simulink model "cyclocopter"  (R2015b)
settings: Solver=VariableStepAuto  SolverMode=SingleTasking  StartTime=0.0  StopTime=100  FixedStep=0.001  RelTol=1e-3
InitFcn:
  | % Update Rates, 50Hz for RC kit
  | fs_servo = 50; %Hz
  | Ts_servo = 1/fs_servo;
  | 
  | % Rates of changes
  | rate = 500; % rad/s per second change
  | rate_p = 2000; % Same for balancing props
  | 
  | % Motor limits
  | limit_high = 8000 * (2 * pi / 60); % rad/s
  | limit_low = 300 * (2 * pi / 60); % rad/s
  | 
  | limit_p_high = 20000 * (2 * pi / 60); % rad/s
  | limit_p_low  = 2000 * (2 * pi / 60);
  | 
  | % Eccentric point limits
  | servo_offset = 0.22;
  | servo_high = pi/4 + servo_offset; %45 deg
  | servo_low = -pi/4 + servo_offset; %45 deg
  | 
  | % Controller Update rate
  | fs = 200; % Hz
  | Ts = 1/fs;
  | 
  | % Constantss
  | g = 9.81; % Gravity
  | 
  | load('cyclorotor_lookup.mat');
values from neighbouring files (symbols this model uses):
  breakpoint_epsilon = [0 0.0175019089336 0.0350038178673 0.0525057268009 0.0700076357346 0.0875095446682 0.105011453602 0.122513362536 0.140015271469 0.157517180403 0.175019089336 0.19252099827 ... (360 elements, 1x360)]    [cyclorotor_lookup.mat]
  breakpoint_omega = [0 5.26229925224 10.5245985045 15.7868977567 21.049197009 26.3114962612 31.5737955135 36.8360947657 42.098394018 47.3606932702 52.6229925224 57.8852917747 ... (200 elements, 1x200)]    [cyclorotor_lookup.mat]
  cyclorotor_lookup = [0 -0.000183077012455 -0.000732308049818 -0.00164769311209 -0.00292923219927 -0.00457692531136 -0.00659077244836 -0.00897077361027 -0.0117169287971 -0.0148292380088 -0.0183077012455 -0.022152318507 ... (432000 elements, 200x360x6)]    [cyclorotor_lookup.mat]
  F = zeros(3, numPoints)    [test_cyclorotor.m]
  r = 0.069    [Cyclorotor.m]
undefined symbols (not defined in the file or in its folder): MIL
libraries: simulink x14, aerolibwind2 x1, aerolibtransform2 x1
settings Model: Creator=freddiesherratt  LastModifiedBy=freddiesherratt
settings DataIOCC: MaxDataPoints=4000  SaveOutput=off  SaveTime=off

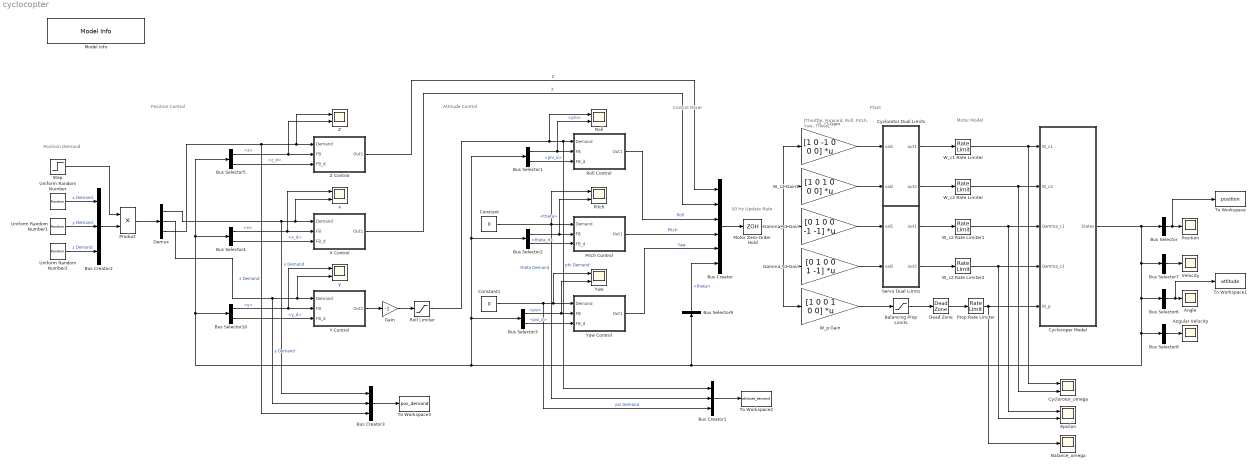
== system cyclocopter ==
  note: Position Demand
  note: Attitude Control
  note: Plant
  note: 50 Hz Update Rate
  note: Motor Model
  note: Control Mixer
  note: [Throttle, Forward, Roll, Pitch, Yaw, Theta]
  note: Position Control
  Angle : Scope
  Angular Velocity : Scope
  Balance_omega : Scope
  Balancing Prop Limits : Saturate  UpperLimit=limit_p_high  LowerLimit=0
  Bus Creator : BusCreator  Inputs=6
  Bus Creator1 : BusCreator  Inputs=3
  Bus Creator2 : BusCreator  Inputs=3
  Bus Creator3 : BusCreator  Inputs=3
  Bus Selector : BusSelector  OutputSignals=x,y,z  OutputAsBus=on
  Bus Selector1 : BusSelector  OutputSignals=phi,phi_d
  Bus Selector10 : BusSelector  OutputSignals=y,y_d
  Bus Selector2 : BusSelector  OutputSignals=theta,theta_d
  Bus Selector3 : BusSelector  OutputSignals=psi,psi_d
  Bus Selector4 : BusSelector  OutputSignals=x,x_d
  Bus Selector5 : BusSelector  OutputSignals=z,z_d
  Bus Selector6 : BusSelector  OutputSignals=phi,theta,psi  OutputAsBus=on
  Bus Selector7 : BusSelector  OutputSignals=x_d,y_d,z_d  OutputAsBus=on
  Bus Selector8 : BusSelector  OutputSignals=phi_d,theta_d,psi_d  OutputAsBus=on
  Bus Selector9 : BusSelector  OutputSignals=theta
  Constant : Constant  Value=0
  Constant1 : Constant  Value=0
  Cyclocoper Model : Subsystem  mask{Ic=0, Im=0, ws=4.5}
      mask prompts: Ic "Ic, Cyclorotor Inertia"; Im "Im, Motor inertia"; ws "ws, wind speed (m/s)"
  Cyclorotor Dual Limits : MATLAB Function  TreatAsAtomicUnit=on  mask{LL=limit_low, UL=limit_high}
      mask prompts: LL "LL, Lower Limit"; UL "UL, Upper Limit"
  Cyclorotor_omega : Scope  NumInputPorts=2
  Dead Zone : DeadZone  LowerValue=0  UpperValue=limit_p_low  SaturateOnIntegerOverflow=on
  Demux : Demux  Outputs=3
  Epsilon : Scope  NumInputPorts=2
  Gain : Gain  Gain=-1
  Gamma_c1 Gain : Gain  Gain=[0 1 0 0 -1 -1]  Multiplication=Matrix(K*u)
  Gamma_c2 Gain : Gain  Gain=[0 1 0 0 1 -1]  Multiplication=Matrix(K*u)
  Model Info : simulink/Model-Wide Utilities/Model Info  Frame=on  DisplayStringWithTags=|  HorizontalTextAlignment=Left  LeftAlignmentValue=0.02  SourceBlockDiagram=cyclocopter  TagMaxNumber=20
      | Last Modified: %<ModifiedDate>
      | By: %<LastModifiedBy>
      | version: %<ModelVersion>
  Motor Zero-Order Hold : ZeroOrderHold  SampleTime=Ts_servo
  Pitch : Scope  NumInputPorts=2
  Pitch Control : Subsystem  mask{P1=18, I1=0, D1=10, P2=25, I2=10, D2=20}
  Position : Scope
  Product : Product
  Prop Rate Limiter : RateLimiter  RisingSlewLimit=rate_p  FallingSlewLimit=-rate_p  SampleTimeMode=inherited  InitialCondition=50
  Roll : Scope  NumInputPorts=2
  Roll Control : Subsystem  mask{P1=10, I1=0, D1=10, P2=7, I2=0.2, D2=0.25}
  Roll Limiter : Saturate  UpperLimit=pi/3  LowerLimit=-pi/3
  Servo Dual Limits : MATLAB Function  TreatAsAtomicUnit=on  mask{LL=servo_low, UL=servo_high}
      mask prompts: LL "LL, Lower Limit"; UL "UL, Upper Limit"
  Step : Step  Time=20  SampleTime=0
  To Workspace : ToWorkspace  VariableName=position  SaveFormat=Timeseries  SampleTime=-1
  To Workspace1 : ToWorkspace  VariableName=attitude  SaveFormat=Timeseries  SampleTime=-1
  To Workspace2 : ToWorkspace  VariableName=attitude_demand  SaveFormat=Timeseries  SampleTime=-1
  To Workspace3 : ToWorkspace  VariableName=pos_demand  SaveFormat=Timeseries  SampleTime=-1
  Uniform Random Number : UniformRandomNumber  Minimum=-3  Maximum=3  SampleTime=10
  Uniform Random Number1 : UniformRandomNumber  Minimum=-3  Maximum=3  Seed=1  SampleTime=10
  Uniform Random Number2 : UniformRandomNumber  Minimum=-3  Maximum=3  Seed=2  SampleTime=10
  Velocity : Scope
  W_c1 Gain : Gain  Gain=[1 0 -1 0 0 0]  Multiplication=Matrix(K*u)
  W_c1 Rate Limiter : RateLimiter  RisingSlewLimit=rate  FallingSlewLimit=-rate
  W_c2 Gain1 : Gain  Gain="[1 0 1  0 0 0]"  Multiplication=Matrix(K*u)
  W_c2 Rate Limiter : RateLimiter  RisingSlewLimit=rate  FallingSlewLimit=-rate
  W_c2 Rate Limiter1 : RateLimiter  RisingSlewLimit=pi  FallingSlewLimit=-pi  InitialCondition=servo_offset
  W_c2 Rate Limiter2 : RateLimiter  RisingSlewLimit=pi  FallingSlewLimit=-pi  InitialCondition=servo_offset
  W_p Gain : Gain  Gain=[1 0 0 1 0 0]  Multiplication=Matrix(K*u)
  X Control : Subsystem  mask{P1=3.2, I1=0, D1=4, P2=0.8, I2=0.2, D2=0.3}
  Y Control : Subsystem  mask{P1=0.2, I1=0, D1=0.55, P2=0.5, I2=0.05, D2=0.15}
  Yaw : Scope  NumInputPorts=2
  Yaw Control : Subsystem  mask{P1=2, I1=0, D1=2, P2=0.4, I2=0.01, D2=0.03}
  Z : Scope  NumInputPorts=2
  Z Control : Subsystem  mask{P1=15, I1=0, D1=15, P2=2.8, I2=1.8, D2=1}
  x : Scope  NumInputPorts=2
  y : Scope  NumInputPorts=2
  wires:
  Bus Selector/1 -> Position/1, To Workspace/1
  Cyclorotor Dual Limits/2(out2) -> W_c2 Rate Limiter/1
  Cyclorotor Dual Limits/1(out1) -> W_c1 Rate Limiter/1
  Motor Zero-Order Hold/1 -> W_c1 Gain/1, W_c2 Gain1/1, W_p Gain/1, Gamma_c2 Gain/1, Gamma_c1 Gain/1
  Bus Creator/1 -> Motor Zero-Order Hold/1
  Roll Control/1(Out1) -> Bus Creator/3  "Roll"
  Z Control/1(Out1) -> Bus Creator/1  "Z"
  Gamma_c1 Gain/1 -> Servo Dual Limits/1(val1)
  Gamma_c2 Gain/1 -> Servo Dual Limits/2(val2)
  Yaw Control/1(Out1) -> Bus Creator/5  "Yaw"
  Pitch Control/1(Out1) -> Bus Creator/4  "Pitch"
  W_c2 Gain1/1 -> Cyclorotor Dual Limits/2(val2)
  W_c1 Gain/1 -> Cyclorotor Dual Limits/1(val1)
  X Control/1(Out1) -> Bus Creator/2  "X"
  Bus Selector5/1 -> Z/2, Z Control/2(FB)  "<z>"
  Bus Selector5/2 -> Z Control/3(FB_d)  "<z_d>"
  Bus Selector4/1 -> x/1, X Control/2(FB)  "<x>"
  Bus Selector4/2 -> X Control/3(FB_d)  "<x_d>"
  Bus Selector1/1 -> Roll/2, Roll Control/2(FB)  "<phi>"
  Bus Selector1/2 -> Roll Control/3(FB_d)  "<phi_d>"
  Bus Selector2/1 -> Pitch/2, Pitch Control/2(FB)  "<theta>"
  Bus Selector2/2 -> Pitch Control/3(FB_d)  "<theta_d>"
  Bus Selector3/1 -> Yaw/2, Yaw Control/2(FB)  "<psi>"
  Bus Selector3/2 -> Yaw Control/3(FB_d)  "<psi_d>"
  Demux/3 -> Bus Creator3/3, Z/1, Z Control/1(Demand)  "z Demand"
  Demux/1 -> Bus Creator3/1, x/2, X Control/1(Demand)  "x Demand"
  Constant/1 -> Pitch/1, Bus Creator1/2, Pitch Control/1(Demand)  "theta Demand"
  Constant1/1 -> Bus Creator1/3, Yaw/1, Yaw Control/1(Demand)  "psi Demand"
  W_c2 Rate Limiter/1 -> Cyclorotor_omega/2, Cyclocoper Model/2(W_c2)
  W_c1 Rate Limiter/1 -> Cyclorotor_omega/1, Cyclocoper Model/1(W_c1)
  Bus Selector6/1 -> Angle/1, To Workspace1/1
  Cyclocoper Model/1(States) -> Bus Selector10/1, Bus Selector4/1, Bus Selector5/1, Bus Selector1/1, Bus Selector2/1, Bus Selector3/1, Bus Selector9/1, Bus Selector8/1, Bus Selector6/1, Bus Selector7/1, Bus Selector/1
  Bus Selector7/1 -> Velocity/1
  Bus Selector8/1 -> Angular Velocity/1
  Bus Selector9/1 -> Bus Creator/6  "<theta>"
  Bus Selector10/1 -> y/1, Y Control/2(FB)  "<y>"
  Bus Selector10/2 -> Y Control/3(FB_d)  "<y_d>"
  Demux/2 -> Bus Creator3/2, y/2, Y Control/1(Demand)  "y Demand"
  Y Control/1(Out1) -> Gain/1
  Gain/1 -> Roll Limiter/1
  Balancing Prop Limits/1 -> Dead Zone/1
  Servo Dual Limits/1(out1) -> W_c2 Rate Limiter1/1
  Servo Dual Limits/2(out2) -> W_c2 Rate Limiter2/1
  W_p Gain/1 -> Balancing Prop Limits/1
  W_c2 Rate Limiter1/1 -> Epsilon/1, Cyclocoper Model/3(Gamma_c1)
  W_c2 Rate Limiter2/1 -> Epsilon/2, Cyclocoper Model/4(Gamma_c2)
  Roll Limiter/1 -> Roll/1, Bus Creator1/1, Roll Control/1(Demand)  "phi Demand"
  Dead Zone/1 -> Prop Rate Limiter/1
  Uniform Random Number2/1 -> Bus Creator2/3  "z Demand"
  Uniform Random Number1/1 -> Bus Creator2/2  "y Demand"
  Uniform Random Number/1 -> Bus Creator2/1  "x Demand"
  Bus Creator2/1 -> Product/2
  Step/1 -> Product/1
  Prop Rate Limiter/1 -> Balance_omega/1, Cyclocoper Model/5(W_p)
  Product/1 -> Demux/1
  Bus Creator1/1 -> To Workspace2/1
  Bus Creator3/1 -> To Workspace3/1

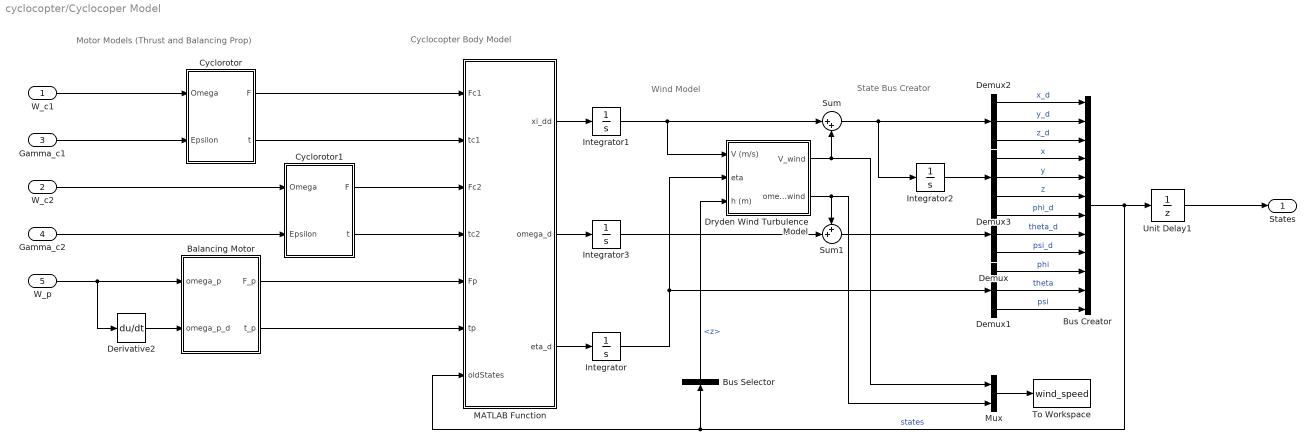
== system cyclocopter/Cyclocoper Model ==
  note: Wind Model
  note: State Bus Creator
  note: Cyclocopter Body Model
  note: Motor Models (Thrust and Balancing Prop)
  W_c1 : Inport
  W_c2 : Inport  Port=2
  Gamma_c1 : Inport  Port=3
  Gamma_c2 : Inport  Port=4
  W_p : Inport  Port=5
  Balancing Motor : MATLAB Function  TreatAsAtomicUnit=on  mask{I_m=Im}
  Bus Creator : BusCreator  Inputs=12
  Bus Selector : BusSelector  OutputSignals=z
  Cyclorotor : Subsystem  mask{I_c=Ic}
      mask prompts: I_c "I_c, Cyclorotor Rotational Inertia"
  Cyclorotor1 : Subsystem  mask{I_c=Ic}
      mask prompts: I_c "I_c, Cyclorotor Rotational Inertia"
  Demux{,1..3} (4 alike) : Demux  Outputs=3
  Derivative2 : Derivative
  Dryden Wind Turbulence Model : Subsystem  mask{ws=ws}
      mask prompts: ws "ws, wind speed (m/s)"
  Integrator{,1..3} (4 alike) : Integrator
  MATLAB Function : MATLAB Function  TreatAsAtomicUnit=on
  Mux : Mux  Inputs=2
  Sum : Sum  Inputs=|++
  Sum1 : Sum  Inputs=++|
  To Workspace : ToWorkspace  VariableName=wind_speed  SaveFormat=Timeseries  SampleTime=-1
  Unit Delay1 : UnitDelay  SampleTime=Ts
  States : Outport
  wires:
  Demux/3 -> Bus Creator/9  "psi_d"
  Demux1/1 -> Bus Creator/10  "phi"
  Balancing Motor/1(F_p) -> MATLAB Function/5(Fp)
  Bus Creator/1 -> Bus Selector/1, MATLAB Function/7(oldStates), Unit Delay1/1  "states"
  Demux3/2 -> Bus Creator/5  "y"
  Demux3/3 -> Bus Creator/6  "z"
  Demux/2 -> Bus Creator/8  "theta_d"
  Demux2/3 -> Bus Creator/3  "z_d"
  Demux3/1 -> Bus Creator/4  "x"
  Demux2/2 -> Bus Creator/2  "y_d"
  Demux2/1 -> Bus Creator/1  "x_d"
  Demux1/3 -> Bus Creator/12  "psi"
  Demux/1 -> Bus Creator/7  "phi_d"
  Demux1/2 -> Bus Creator/11  "theta"
  W_p/1 -> Derivative2/1, Balancing Motor/1(omega_p)
  Gamma_c2/1 -> Cyclorotor1/2(Epsilon)
  W_c2/1 -> Cyclorotor1/1(Omega)
  Balancing Motor/2(t_p) -> MATLAB Function/6(tp)
  MATLAB Function/1(xi_dd) -> Integrator1/1
  Derivative2/1 -> Balancing Motor/2(omega_p_d)
  Integrator1/1 -> Sum/1, Dryden Wind Turbulence Model/1(V (m/s))
  Integrator2/1 -> Demux3/1
  Unit Delay1/1 -> States/1
  Integrator/1 -> Demux1/1, Dryden Wind Turbulence Model/2(eta)
  Sum/1 -> Integrator2/1, Demux2/1
  Integrator3/1 -> Sum1/2
  Sum1/1 -> Demux/1
  Bus Selector/1 -> Dryden Wind Turbulence Model/3(h (m))  "<z>"
  Dryden Wind Turbulence Model/2(omega_wind) -> Sum1/1, Mux/2
  MATLAB Function/2(omega_d) -> Integrator3/1
  MATLAB Function/3(eta_d) -> Integrator/1
  W_c1/1 -> Cyclorotor/1(Omega)
  Gamma_c1/1 -> Cyclorotor/2(Epsilon)
  Cyclorotor/1(F) -> MATLAB Function/1(Fc1)
  Cyclorotor/2(t) -> MATLAB Function/2(tc1)
  Cyclorotor1/2(t) -> MATLAB Function/4(tc2)
  Cyclorotor1/1(F) -> MATLAB Function/3(Fc2)
  Dryden Wind Turbulence Model/1(V_wind) -> Mux/1, Sum/2
  Mux/1 -> To Workspace/1

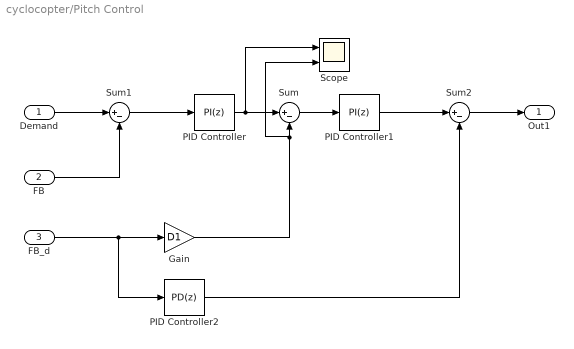
== system cyclocopter/Pitch Control ==
  Demand : Inport
  FB : Inport  Port=2
  FB_d : Inport  Port=3
  Gain : Gain  Gain=D1
  PID Controller : simulink/Continuous/PID Controller  Controller=PI  TimeDomain=Discrete-time  SampleTime=Ts  IntegratorMethod=Forward Euler  FilterMethod=Forward Euler  Form=Parallel  UseFilter=on  ControllerParametersSource=internal  P=P1  I=I1  D=0  N=100  InitialConditionSource=internal  InitialConditionForIntegrator=0  InitialConditionForFilter=0  ExternalReset=none  LimitOutput=off  UpperSaturationLimit=inf  LowerSaturationLimit=-inf  LinearizeAsGain=on  AntiWindupMode=none  Kb=1  TrackingMode=off  Kt=1  PParamMin=[]  PParamMax=[]  IParamMin=[]  IParamMax=[]  DParamMin=[]  DParamMax=[]  NParamMin=[]  NParamMax=[]  KbParamMin=[]  KbParamMax=[]  KtParamMin=[]  KtParamMax=[]  POutMin=[]  POutMax=[]  IOutMin=[]  IOutMax=[]  DOutMin=[]  DOutMax=[]  NOutMin=[]  NOutMax=[]  KbOutMin=[]  KbOutMax=[]  KtOutMin=[]  KtOutMax=[]  IntegratorOutMin=[]  IntegratorOutMax=[]  FilterOutMin=[]  FilterOutMax=[]  SumOutMin=[]  SumOutMax=[]  SumI1OutMin=[]  SumI1OutMax=[]  SumI2OutMin=[]  SumI2OutMax=[]  SumI3OutMin=[]  SumI3OutMax=[]  SumDOutMin=[]  SumDOutMax=[]  SaturationOutMin=[]  SaturationOutMax=[]  IntegratorContinuousStateAttributes=''  IntegratorStateMustResolveToSignalObject=off  IntegratorRTWStateStorageClass=Auto  FilterContinuousStateAttributes=''  FilterStateMustResolveToSignalObject=off  FilterRTWStateStorageClass=Auto  DifferentiatorICPrevScaledInput=0  DifferentiatorOutMin=[]  DifferentiatorOutMax=[]
  PID Controller1 : simulink/Continuous/PID Controller  Controller=PI  TimeDomain=Discrete-time  SampleTime=Ts  IntegratorMethod=Forward Euler  FilterMethod=Forward Euler  Form=Parallel  UseFilter=on  ControllerParametersSource=internal  P=P2  I=I2  D=0  N=100  InitialConditionSource=internal  InitialConditionForIntegrator=0  InitialConditionForFilter=0  ExternalReset=none  LimitOutput=off  UpperSaturationLimit=inf  LowerSaturationLimit=-inf  LinearizeAsGain=on  AntiWindupMode=none  Kb=1  TrackingMode=off  Kt=1  PParamMin=[]  PParamMax=[]  IParamMin=[]  IParamMax=[]  DParamMin=[]  DParamMax=[]  NParamMin=[]  NParamMax=[]  KbParamMin=[]  KbParamMax=[]  KtParamMin=[]  KtParamMax=[]  POutMin=[]  POutMax=[]  IOutMin=[]  IOutMax=[]  DOutMin=[]  DOutMax=[]  NOutMin=[]  NOutMax=[]  KbOutMin=[]  KbOutMax=[]  KtOutMin=[]  KtOutMax=[]  IntegratorOutMin=[]  IntegratorOutMax=[]  FilterOutMin=[]  FilterOutMax=[]  SumOutMin=[]  SumOutMax=[]  SumI1OutMin=[]  SumI1OutMax=[]  SumI2OutMin=[]  SumI2OutMax=[]  SumI3OutMin=[]  SumI3OutMax=[]  SumDOutMin=[]  SumDOutMax=[]  SaturationOutMin=[]  SaturationOutMax=[]  IntegratorContinuousStateAttributes=''  IntegratorStateMustResolveToSignalObject=off  IntegratorRTWStateStorageClass=Auto  FilterContinuousStateAttributes=''  FilterStateMustResolveToSignalObject=off  FilterRTWStateStorageClass=Auto  DifferentiatorICPrevScaledInput=0  DifferentiatorOutMin=[]  DifferentiatorOutMax=[]
  PID Controller2 : simulink/Continuous/PID Controller  Controller=PD  TimeDomain=Discrete-time  SampleTime=Ts  IntegratorMethod=Forward Euler  FilterMethod=Forward Euler  Form=Parallel  UseFilter=on  ControllerParametersSource=internal  P=0  I=I2  D=D2  N=100  InitialConditionSource=internal  InitialConditionForIntegrator=0  InitialConditionForFilter=0  ExternalReset=none  LimitOutput=off  UpperSaturationLimit=inf  LowerSaturationLimit=-inf  LinearizeAsGain=on  AntiWindupMode=none  Kb=1  TrackingMode=off  Kt=1  PParamMin=[]  PParamMax=[]  IParamMin=[]  IParamMax=[]  DParamMin=[]  DParamMax=[]  NParamMin=[]  NParamMax=[]  KbParamMin=[]  KbParamMax=[]  KtParamMin=[]  KtParamMax=[]  POutMin=[]  POutMax=[]  IOutMin=[]  IOutMax=[]  DOutMin=[]  DOutMax=[]  NOutMin=[]  NOutMax=[]  KbOutMin=[]  KbOutMax=[]  KtOutMin=[]  KtOutMax=[]  IntegratorOutMin=[]  IntegratorOutMax=[]  FilterOutMin=[]  FilterOutMax=[]  SumOutMin=[]  SumOutMax=[]  SumI1OutMin=[]  SumI1OutMax=[]  SumI2OutMin=[]  SumI2OutMax=[]  SumI3OutMin=[]  SumI3OutMax=[]  SumDOutMin=[]  SumDOutMax=[]  SaturationOutMin=[]  SaturationOutMax=[]  IntegratorContinuousStateAttributes=''  IntegratorStateMustResolveToSignalObject=off  IntegratorRTWStateStorageClass=Auto  FilterContinuousStateAttributes=''  FilterStateMustResolveToSignalObject=off  FilterRTWStateStorageClass=Auto  DifferentiatorICPrevScaledInput=0  DifferentiatorOutMin=[]  DifferentiatorOutMax=[]
  Scope : Scope  NumInputPorts=2
  Sum : Sum  Inputs=|+-
  Sum1 : Sum  Inputs=|+-
  Sum2 : Sum  Inputs=|+-
  Out1 : Outport
  wires:
  Sum2/1 -> Out1/1
  PID Controller2/1 -> Sum2/2
  Gain/1 -> Scope/2, Sum/2
  PID Controller1/1 -> Sum2/1
  PID Controller/1 -> Scope/1, Sum/1
  FB_d/1 -> PID Controller2/1, Gain/1
  Sum1/1 -> PID Controller/1
  Demand/1 -> Sum1/1
  FB/1 -> Sum1/2
  Sum/1 -> PID Controller1/1

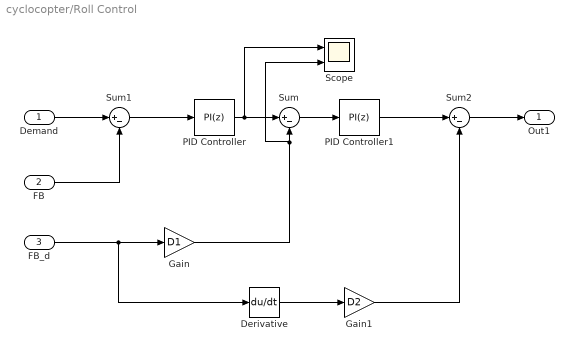
== system cyclocopter/Roll Control ==
  Demand : Inport
  FB : Inport  Port=2
  FB_d : Inport  Port=3
  Derivative : Derivative
  Gain : Gain  Gain=D1
  Gain1 : Gain  Gain=D2
  PID Controller : simulink/Continuous/PID Controller  Controller=PI  TimeDomain=Discrete-time  SampleTime=Ts  IntegratorMethod=Forward Euler  FilterMethod=Forward Euler  Form=Parallel  UseFilter=on  ControllerParametersSource=internal  P=P1  I=I1  D=0  N=100  InitialConditionSource=internal  InitialConditionForIntegrator=0  InitialConditionForFilter=0  ExternalReset=none  LimitOutput=off  UpperSaturationLimit=inf  LowerSaturationLimit=-inf  LinearizeAsGain=on  AntiWindupMode=none  Kb=1  TrackingMode=off  Kt=1  PParamMin=[]  PParamMax=[]  IParamMin=[]  IParamMax=[]  DParamMin=[]  DParamMax=[]  NParamMin=[]  NParamMax=[]  KbParamMin=[]  KbParamMax=[]  KtParamMin=[]  KtParamMax=[]  POutMin=[]  POutMax=[]  IOutMin=[]  IOutMax=[]  DOutMin=[]  DOutMax=[]  NOutMin=[]  NOutMax=[]  KbOutMin=[]  KbOutMax=[]  KtOutMin=[]  KtOutMax=[]  IntegratorOutMin=[]  IntegratorOutMax=[]  FilterOutMin=[]  FilterOutMax=[]  SumOutMin=[]  SumOutMax=[]  SumI1OutMin=[]  SumI1OutMax=[]  SumI2OutMin=[]  SumI2OutMax=[]  SumI3OutMin=[]  SumI3OutMax=[]  SumDOutMin=[]  SumDOutMax=[]  SaturationOutMin=[]  SaturationOutMax=[]  IntegratorContinuousStateAttributes=''  IntegratorStateMustResolveToSignalObject=off  IntegratorRTWStateStorageClass=Auto  FilterContinuousStateAttributes=''  FilterStateMustResolveToSignalObject=off  FilterRTWStateStorageClass=Auto  DifferentiatorICPrevScaledInput=0  DifferentiatorOutMin=[]  DifferentiatorOutMax=[]
  PID Controller1 : simulink/Continuous/PID Controller  Controller=PI  TimeDomain=Discrete-time  SampleTime=Ts  IntegratorMethod=Forward Euler  FilterMethod=Forward Euler  Form=Parallel  UseFilter=on  ControllerParametersSource=internal  P=P2  I=I2  D=0  N=100  InitialConditionSource=internal  InitialConditionForIntegrator=0  InitialConditionForFilter=0  ExternalReset=none  LimitOutput=off  UpperSaturationLimit=inf  LowerSaturationLimit=-inf  LinearizeAsGain=on  AntiWindupMode=none  Kb=1  TrackingMode=off  Kt=1  PParamMin=[]  PParamMax=[]  IParamMin=[]  IParamMax=[]  DParamMin=[]  DParamMax=[]  NParamMin=[]  NParamMax=[]  KbParamMin=[]  KbParamMax=[]  KtParamMin=[]  KtParamMax=[]  POutMin=[]  POutMax=[]  IOutMin=[]  IOutMax=[]  DOutMin=[]  DOutMax=[]  NOutMin=[]  NOutMax=[]  KbOutMin=[]  KbOutMax=[]  KtOutMin=[]  KtOutMax=[]  IntegratorOutMin=[]  IntegratorOutMax=[]  FilterOutMin=[]  FilterOutMax=[]  SumOutMin=[]  SumOutMax=[]  SumI1OutMin=[]  SumI1OutMax=[]  SumI2OutMin=[]  SumI2OutMax=[]  SumI3OutMin=[]  SumI3OutMax=[]  SumDOutMin=[]  SumDOutMax=[]  SaturationOutMin=[]  SaturationOutMax=[]  IntegratorContinuousStateAttributes=''  IntegratorStateMustResolveToSignalObject=off  IntegratorRTWStateStorageClass=Auto  FilterContinuousStateAttributes=''  FilterStateMustResolveToSignalObject=off  FilterRTWStateStorageClass=Auto  DifferentiatorICPrevScaledInput=0  DifferentiatorOutMin=[]  DifferentiatorOutMax=[]
  Scope : Scope  NumInputPorts=2
  Sum : Sum  Inputs=|+-
  Sum1 : Sum  Inputs=|+-
  Sum2 : Sum  Inputs=|+-
  Out1 : Outport
  wires:
  Sum/1 -> PID Controller1/1
  FB/1 -> Sum1/2
  Demand/1 -> Sum1/1
  Sum1/1 -> PID Controller/1
  FB_d/1 -> Derivative/1, Gain/1
  PID Controller/1 -> Scope/1, Sum/1
  PID Controller1/1 -> Sum2/1
  Gain/1 -> Scope/2, Sum/2
  Gain1/1 -> Sum2/2
  Derivative/1 -> Gain1/1
  Sum2/1 -> Out1/1

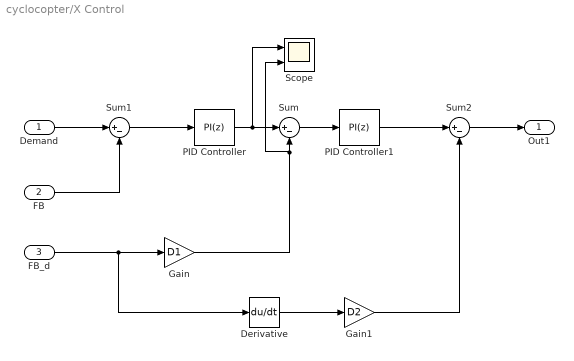
== system cyclocopter/X Control ==
  Demand : Inport
  FB : Inport  Port=2
  FB_d : Inport  Port=3
  Derivative : Derivative
  Gain : Gain  Gain=D1
  Gain1 : Gain  Gain=D2
  PID Controller : simulink/Continuous/PID Controller  Controller=PI  TimeDomain=Discrete-time  SampleTime=Ts  IntegratorMethod=Forward Euler  FilterMethod=Forward Euler  Form=Parallel  UseFilter=on  ControllerParametersSource=internal  P=P1  I=I1  D=0  N=100  InitialConditionSource=internal  InitialConditionForIntegrator=0  InitialConditionForFilter=0  ExternalReset=none  LimitOutput=off  UpperSaturationLimit=inf  LowerSaturationLimit=-inf  LinearizeAsGain=on  AntiWindupMode=none  Kb=1  TrackingMode=off  Kt=1  PParamMin=[]  PParamMax=[]  IParamMin=[]  IParamMax=[]  DParamMin=[]  DParamMax=[]  NParamMin=[]  NParamMax=[]  KbParamMin=[]  KbParamMax=[]  KtParamMin=[]  KtParamMax=[]  POutMin=[]  POutMax=[]  IOutMin=[]  IOutMax=[]  DOutMin=[]  DOutMax=[]  NOutMin=[]  NOutMax=[]  KbOutMin=[]  KbOutMax=[]  KtOutMin=[]  KtOutMax=[]  IntegratorOutMin=[]  IntegratorOutMax=[]  FilterOutMin=[]  FilterOutMax=[]  SumOutMin=[]  SumOutMax=[]  SumI1OutMin=[]  SumI1OutMax=[]  SumI2OutMin=[]  SumI2OutMax=[]  SumI3OutMin=[]  SumI3OutMax=[]  SumDOutMin=[]  SumDOutMax=[]  SaturationOutMin=[]  SaturationOutMax=[]  IntegratorContinuousStateAttributes=''  IntegratorStateMustResolveToSignalObject=off  IntegratorRTWStateStorageClass=Auto  FilterContinuousStateAttributes=''  FilterStateMustResolveToSignalObject=off  FilterRTWStateStorageClass=Auto  DifferentiatorICPrevScaledInput=0  DifferentiatorOutMin=[]  DifferentiatorOutMax=[]
  PID Controller1 : simulink/Continuous/PID Controller  Controller=PI  TimeDomain=Discrete-time  SampleTime=Ts  IntegratorMethod=Forward Euler  FilterMethod=Forward Euler  Form=Parallel  UseFilter=on  ControllerParametersSource=internal  P=P2  I=I2  D=0  N=100  InitialConditionSource=internal  InitialConditionForIntegrator=0  InitialConditionForFilter=0  ExternalReset=none  LimitOutput=off  UpperSaturationLimit=inf  LowerSaturationLimit=-inf  LinearizeAsGain=on  AntiWindupMode=none  Kb=1  TrackingMode=off  Kt=1  PParamMin=[]  PParamMax=[]  IParamMin=[]  IParamMax=[]  DParamMin=[]  DParamMax=[]  NParamMin=[]  NParamMax=[]  KbParamMin=[]  KbParamMax=[]  KtParamMin=[]  KtParamMax=[]  POutMin=[]  POutMax=[]  IOutMin=[]  IOutMax=[]  DOutMin=[]  DOutMax=[]  NOutMin=[]  NOutMax=[]  KbOutMin=[]  KbOutMax=[]  KtOutMin=[]  KtOutMax=[]  IntegratorOutMin=[]  IntegratorOutMax=[]  FilterOutMin=[]  FilterOutMax=[]  SumOutMin=[]  SumOutMax=[]  SumI1OutMin=[]  SumI1OutMax=[]  SumI2OutMin=[]  SumI2OutMax=[]  SumI3OutMin=[]  SumI3OutMax=[]  SumDOutMin=[]  SumDOutMax=[]  SaturationOutMin=[]  SaturationOutMax=[]  IntegratorContinuousStateAttributes=''  IntegratorStateMustResolveToSignalObject=off  IntegratorRTWStateStorageClass=Auto  FilterContinuousStateAttributes=''  FilterStateMustResolveToSignalObject=off  FilterRTWStateStorageClass=Auto  DifferentiatorICPrevScaledInput=0  DifferentiatorOutMin=[]  DifferentiatorOutMax=[]
  Scope : Scope  NumInputPorts=2
  Sum : Sum  Inputs=|+-
  Sum1 : Sum  Inputs=|+-
  Sum2 : Sum  Inputs=|+-
  Out1 : Outport
  wires:
  Sum2/1 -> Out1/1
  Derivative/1 -> Gain1/1
  Gain1/1 -> Sum2/2
  Gain/1 -> Scope/2, Sum/2
  PID Controller1/1 -> Sum2/1
  PID Controller/1 -> Scope/1, Sum/1
  FB_d/1 -> Gain/1, Derivative/1
  Sum1/1 -> PID Controller/1
  Demand/1 -> Sum1/1
  FB/1 -> Sum1/2
  Sum/1 -> PID Controller1/1

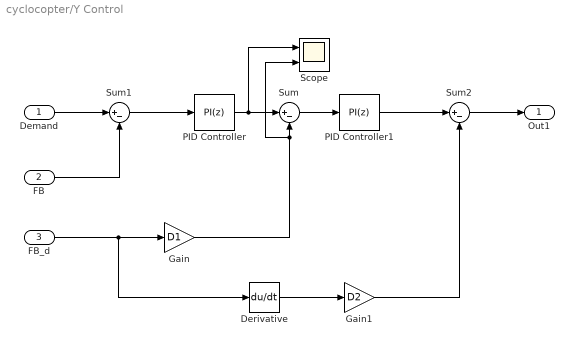
== system cyclocopter/Y Control ==
  Demand : Inport
  FB : Inport  Port=2
  FB_d : Inport  Port=3
  Derivative : Derivative
  Gain : Gain  Gain=D1
  Gain1 : Gain  Gain=D2
  PID Controller : simulink/Continuous/PID Controller  Controller=PI  TimeDomain=Discrete-time  SampleTime=Ts  IntegratorMethod=Forward Euler  FilterMethod=Forward Euler  Form=Parallel  UseFilter=on  ControllerParametersSource=internal  P=P1  I=I1  D=0  N=100  InitialConditionSource=internal  InitialConditionForIntegrator=0  InitialConditionForFilter=0  ExternalReset=none  LimitOutput=off  UpperSaturationLimit=inf  LowerSaturationLimit=-inf  LinearizeAsGain=on  AntiWindupMode=none  Kb=1  TrackingMode=off  Kt=1  PParamMin=[]  PParamMax=[]  IParamMin=[]  IParamMax=[]  DParamMin=[]  DParamMax=[]  NParamMin=[]  NParamMax=[]  KbParamMin=[]  KbParamMax=[]  KtParamMin=[]  KtParamMax=[]  POutMin=[]  POutMax=[]  IOutMin=[]  IOutMax=[]  DOutMin=[]  DOutMax=[]  NOutMin=[]  NOutMax=[]  KbOutMin=[]  KbOutMax=[]  KtOutMin=[]  KtOutMax=[]  IntegratorOutMin=[]  IntegratorOutMax=[]  FilterOutMin=[]  FilterOutMax=[]  SumOutMin=[]  SumOutMax=[]  SumI1OutMin=[]  SumI1OutMax=[]  SumI2OutMin=[]  SumI2OutMax=[]  SumI3OutMin=[]  SumI3OutMax=[]  SumDOutMin=[]  SumDOutMax=[]  SaturationOutMin=[]  SaturationOutMax=[]  IntegratorContinuousStateAttributes=''  IntegratorStateMustResolveToSignalObject=off  IntegratorRTWStateStorageClass=Auto  FilterContinuousStateAttributes=''  FilterStateMustResolveToSignalObject=off  FilterRTWStateStorageClass=Auto  DifferentiatorICPrevScaledInput=0  DifferentiatorOutMin=[]  DifferentiatorOutMax=[]
  PID Controller1 : simulink/Continuous/PID Controller  Controller=PI  TimeDomain=Discrete-time  SampleTime=Ts  IntegratorMethod=Forward Euler  FilterMethod=Forward Euler  Form=Parallel  UseFilter=on  ControllerParametersSource=internal  P=P2  I=I2  D=0  N=100  InitialConditionSource=internal  InitialConditionForIntegrator=0  InitialConditionForFilter=0  ExternalReset=none  LimitOutput=off  UpperSaturationLimit=inf  LowerSaturationLimit=-inf  LinearizeAsGain=on  AntiWindupMode=none  Kb=1  TrackingMode=off  Kt=1  PParamMin=[]  PParamMax=[]  IParamMin=[]  IParamMax=[]  DParamMin=[]  DParamMax=[]  NParamMin=[]  NParamMax=[]  KbParamMin=[]  KbParamMax=[]  KtParamMin=[]  KtParamMax=[]  POutMin=[]  POutMax=[]  IOutMin=[]  IOutMax=[]  DOutMin=[]  DOutMax=[]  NOutMin=[]  NOutMax=[]  KbOutMin=[]  KbOutMax=[]  KtOutMin=[]  KtOutMax=[]  IntegratorOutMin=[]  IntegratorOutMax=[]  FilterOutMin=[]  FilterOutMax=[]  SumOutMin=[]  SumOutMax=[]  SumI1OutMin=[]  SumI1OutMax=[]  SumI2OutMin=[]  SumI2OutMax=[]  SumI3OutMin=[]  SumI3OutMax=[]  SumDOutMin=[]  SumDOutMax=[]  SaturationOutMin=[]  SaturationOutMax=[]  IntegratorContinuousStateAttributes=''  IntegratorStateMustResolveToSignalObject=off  IntegratorRTWStateStorageClass=Auto  FilterContinuousStateAttributes=''  FilterStateMustResolveToSignalObject=off  FilterRTWStateStorageClass=Auto  DifferentiatorICPrevScaledInput=0  DifferentiatorOutMin=[]  DifferentiatorOutMax=[]
  Scope : Scope  NumInputPorts=2
  Sum : Sum  Inputs=|+-
  Sum1 : Sum  Inputs=|+-
  Sum2 : Sum  Inputs=|+-
  Out1 : Outport
  wires:
  Sum/1 -> PID Controller1/1
  FB/1 -> Sum1/2
  Demand/1 -> Sum1/1
  Sum1/1 -> PID Controller/1
  FB_d/1 -> Derivative/1, Gain/1
  PID Controller/1 -> Scope/1, Sum/1
  PID Controller1/1 -> Sum2/1
  Gain/1 -> Scope/2, Sum/2
  Gain1/1 -> Sum2/2
  Derivative/1 -> Gain1/1
  Sum2/1 -> Out1/1

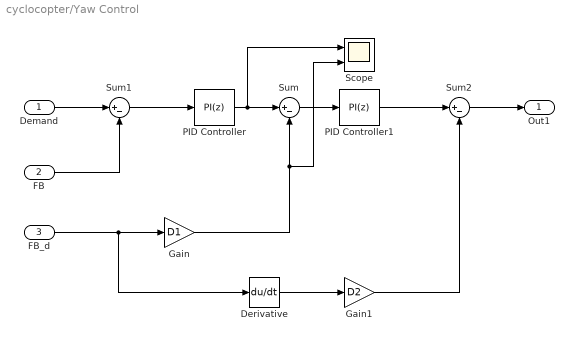
== system cyclocopter/Yaw Control ==
  Demand : Inport
  FB : Inport  Port=2
  FB_d : Inport  Port=3
  Derivative : Derivative
  Gain : Gain  Gain=D1
  Gain1 : Gain  Gain=D2
  PID Controller : simulink/Continuous/PID Controller  Controller=PI  TimeDomain=Discrete-time  SampleTime=Ts  IntegratorMethod=Forward Euler  FilterMethod=Forward Euler  Form=Parallel  UseFilter=on  ControllerParametersSource=internal  P=P1  I=I1  D=0  N=100  InitialConditionSource=internal  InitialConditionForIntegrator=0  InitialConditionForFilter=0  ExternalReset=none  LimitOutput=off  UpperSaturationLimit=inf  LowerSaturationLimit=-inf  LinearizeAsGain=on  AntiWindupMode=none  Kb=1  TrackingMode=off  Kt=1  PParamMin=[]  PParamMax=[]  IParamMin=[]  IParamMax=[]  DParamMin=[]  DParamMax=[]  NParamMin=[]  NParamMax=[]  KbParamMin=[]  KbParamMax=[]  KtParamMin=[]  KtParamMax=[]  POutMin=[]  POutMax=[]  IOutMin=[]  IOutMax=[]  DOutMin=[]  DOutMax=[]  NOutMin=[]  NOutMax=[]  KbOutMin=[]  KbOutMax=[]  KtOutMin=[]  KtOutMax=[]  IntegratorOutMin=[]  IntegratorOutMax=[]  FilterOutMin=[]  FilterOutMax=[]  SumOutMin=[]  SumOutMax=[]  SumI1OutMin=[]  SumI1OutMax=[]  SumI2OutMin=[]  SumI2OutMax=[]  SumI3OutMin=[]  SumI3OutMax=[]  SumDOutMin=[]  SumDOutMax=[]  SaturationOutMin=[]  SaturationOutMax=[]  IntegratorContinuousStateAttributes=''  IntegratorStateMustResolveToSignalObject=off  IntegratorRTWStateStorageClass=Auto  FilterContinuousStateAttributes=''  FilterStateMustResolveToSignalObject=off  FilterRTWStateStorageClass=Auto  DifferentiatorICPrevScaledInput=0  DifferentiatorOutMin=[]  DifferentiatorOutMax=[]
  PID Controller1 : simulink/Continuous/PID Controller  Controller=PI  TimeDomain=Discrete-time  SampleTime=Ts  IntegratorMethod=Forward Euler  FilterMethod=Forward Euler  Form=Parallel  UseFilter=on  ControllerParametersSource=internal  P=P2  I=I2  D=0  N=100  InitialConditionSource=internal  InitialConditionForIntegrator=0  InitialConditionForFilter=0  ExternalReset=none  LimitOutput=off  UpperSaturationLimit=inf  LowerSaturationLimit=-inf  LinearizeAsGain=on  AntiWindupMode=none  Kb=1  TrackingMode=off  Kt=1  PParamMin=[]  PParamMax=[]  IParamMin=[]  IParamMax=[]  DParamMin=[]  DParamMax=[]  NParamMin=[]  NParamMax=[]  KbParamMin=[]  KbParamMax=[]  KtParamMin=[]  KtParamMax=[]  POutMin=[]  POutMax=[]  IOutMin=[]  IOutMax=[]  DOutMin=[]  DOutMax=[]  NOutMin=[]  NOutMax=[]  KbOutMin=[]  KbOutMax=[]  KtOutMin=[]  KtOutMax=[]  IntegratorOutMin=[]  IntegratorOutMax=[]  FilterOutMin=[]  FilterOutMax=[]  SumOutMin=[]  SumOutMax=[]  SumI1OutMin=[]  SumI1OutMax=[]  SumI2OutMin=[]  SumI2OutMax=[]  SumI3OutMin=[]  SumI3OutMax=[]  SumDOutMin=[]  SumDOutMax=[]  SaturationOutMin=[]  SaturationOutMax=[]  IntegratorContinuousStateAttributes=''  IntegratorStateMustResolveToSignalObject=off  IntegratorRTWStateStorageClass=Auto  FilterContinuousStateAttributes=''  FilterStateMustResolveToSignalObject=off  FilterRTWStateStorageClass=Auto  DifferentiatorICPrevScaledInput=0  DifferentiatorOutMin=[]  DifferentiatorOutMax=[]
  Scope : Scope  NumInputPorts=2
  Sum : Sum  Inputs=|+-
  Sum1 : Sum  Inputs=|+-
  Sum2 : Sum  Inputs=|+-
  Out1 : Outport
  wires:
  Sum/1 -> PID Controller1/1
  FB/1 -> Sum1/2
  Demand/1 -> Sum1/1
  Sum1/1 -> PID Controller/1
  FB_d/1 -> Derivative/1, Gain/1
  PID Controller/1 -> Scope/1, Sum/1
  PID Controller1/1 -> Sum2/1
  Gain/1 -> Scope/2, Sum/2
  Gain1/1 -> Sum2/2
  Derivative/1 -> Gain1/1
  Sum2/1 -> Out1/1

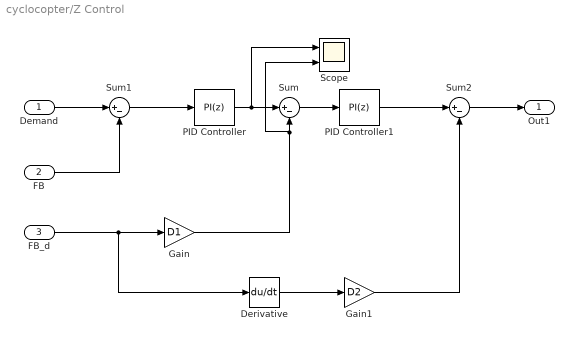
== system cyclocopter/Z Control ==
  Demand : Inport
  FB : Inport  Port=2
  FB_d : Inport  Port=3
  Derivative : Derivative
  Gain : Gain  Gain=D1
  Gain1 : Gain  Gain=D2
  PID Controller : simulink/Continuous/PID Controller  Controller=PI  TimeDomain=Discrete-time  SampleTime=Ts  IntegratorMethod=Forward Euler  FilterMethod=Forward Euler  Form=Parallel  UseFilter=on  ControllerParametersSource=internal  P=P1  I=I1  D=0  N=100  InitialConditionSource=internal  InitialConditionForIntegrator=0  InitialConditionForFilter=0  ExternalReset=none  LimitOutput=off  UpperSaturationLimit=inf  LowerSaturationLimit=-inf  LinearizeAsGain=on  AntiWindupMode=none  Kb=1  TrackingMode=off  Kt=1  PParamMin=[]  PParamMax=[]  IParamMin=[]  IParamMax=[]  DParamMin=[]  DParamMax=[]  NParamMin=[]  NParamMax=[]  KbParamMin=[]  KbParamMax=[]  KtParamMin=[]  KtParamMax=[]  POutMin=[]  POutMax=[]  IOutMin=[]  IOutMax=[]  DOutMin=[]  DOutMax=[]  NOutMin=[]  NOutMax=[]  KbOutMin=[]  KbOutMax=[]  KtOutMin=[]  KtOutMax=[]  IntegratorOutMin=[]  IntegratorOutMax=[]  FilterOutMin=[]  FilterOutMax=[]  SumOutMin=[]  SumOutMax=[]  SumI1OutMin=[]  SumI1OutMax=[]  SumI2OutMin=[]  SumI2OutMax=[]  SumI3OutMin=[]  SumI3OutMax=[]  SumDOutMin=[]  SumDOutMax=[]  SaturationOutMin=[]  SaturationOutMax=[]  IntegratorContinuousStateAttributes=''  IntegratorStateMustResolveToSignalObject=off  IntegratorRTWStateStorageClass=Auto  FilterContinuousStateAttributes=''  FilterStateMustResolveToSignalObject=off  FilterRTWStateStorageClass=Auto  DifferentiatorICPrevScaledInput=0  DifferentiatorOutMin=[]  DifferentiatorOutMax=[]
  PID Controller1 : simulink/Continuous/PID Controller  Controller=PI  TimeDomain=Discrete-time  SampleTime=Ts  IntegratorMethod=Forward Euler  FilterMethod=Forward Euler  Form=Parallel  UseFilter=on  ControllerParametersSource=internal  P=P2  I=I2  D=0  N=100  InitialConditionSource=internal  InitialConditionForIntegrator=0  InitialConditionForFilter=0  ExternalReset=none  LimitOutput=off  UpperSaturationLimit=inf  LowerSaturationLimit=-inf  LinearizeAsGain=on  AntiWindupMode=none  Kb=1  TrackingMode=off  Kt=1  PParamMin=[]  PParamMax=[]  IParamMin=[]  IParamMax=[]  DParamMin=[]  DParamMax=[]  NParamMin=[]  NParamMax=[]  KbParamMin=[]  KbParamMax=[]  KtParamMin=[]  KtParamMax=[]  POutMin=[]  POutMax=[]  IOutMin=[]  IOutMax=[]  DOutMin=[]  DOutMax=[]  NOutMin=[]  NOutMax=[]  KbOutMin=[]  KbOutMax=[]  KtOutMin=[]  KtOutMax=[]  IntegratorOutMin=[]  IntegratorOutMax=[]  FilterOutMin=[]  FilterOutMax=[]  SumOutMin=[]  SumOutMax=[]  SumI1OutMin=[]  SumI1OutMax=[]  SumI2OutMin=[]  SumI2OutMax=[]  SumI3OutMin=[]  SumI3OutMax=[]  SumDOutMin=[]  SumDOutMax=[]  SaturationOutMin=[]  SaturationOutMax=[]  IntegratorContinuousStateAttributes=''  IntegratorStateMustResolveToSignalObject=off  IntegratorRTWStateStorageClass=Auto  FilterContinuousStateAttributes=''  FilterStateMustResolveToSignalObject=off  FilterRTWStateStorageClass=Auto  DifferentiatorICPrevScaledInput=0  DifferentiatorOutMin=[]  DifferentiatorOutMax=[]
  Scope : Scope  NumInputPorts=2
  Sum : Sum  Inputs=|+-
  Sum1 : Sum  Inputs=|+-
  Sum2 : Sum  Inputs=|+-
  Out1 : Outport
  wires:
  Sum/1 -> PID Controller1/1
  FB/1 -> Sum1/2
  Demand/1 -> Sum1/1
  Sum1/1 -> PID Controller/1
  FB_d/1 -> Derivative/1, Gain/1
  PID Controller/1 -> Scope/1, Sum/1
  PID Controller1/1 -> Sum2/1
  Gain/1 -> Scope/2, Sum/2
  Gain1/1 -> Sum2/2
  Derivative/1 -> Gain1/1
  Sum2/1 -> Out1/1

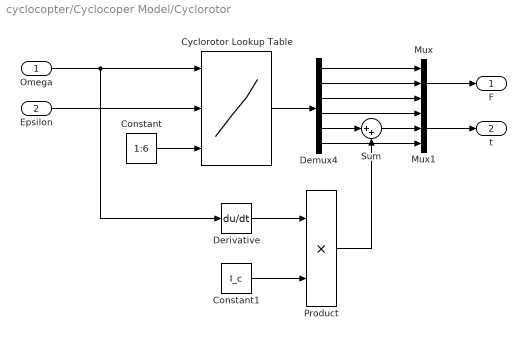
== system cyclocopter/Cyclocoper Model/Cyclorotor ==
  Omega : Inport
  Epsilon : Inport  Port=2
  Constant : Constant  Value=1:6
  Constant1 : Constant  Value=I_c
  Cyclorotor Lookup Table : Lookup_n-D  NumberOfTableDimensions=3  BreakpointsForDimension1=breakpoint_omega  BreakpointsForDimension2=breakpoint_epsilon  BreakpointsForDimension3=[1:6]  Table=cyclorotor_lookup  InternalRulePriority=Speed  OutDataTypeStr=double  RndMeth=Simplest  InputSameDT=on
  Demux4 : Demux  Outputs=6
  Derivative : Derivative
  Mux : Mux  Inputs=3
  Mux1 : Mux  Inputs=3
  Product : Product
  Sum : Sum  Inputs=|++
  F : Outport
  t : Outport  Port=2
  wires:
  Cyclorotor Lookup Table/1 -> Demux4/1
  Mux/1 -> F/1
  Epsilon/1 -> Cyclorotor Lookup Table/2
  Omega/1 -> Derivative/1, Cyclorotor Lookup Table/1
  Mux1/1 -> t/1
  Demux4/5 -> Sum/1
  Demux4/4 -> Mux1/1
  Demux4/6 -> Mux1/3
  Demux4/3 -> Mux/3
  Demux4/2 -> Mux/2
  Constant/1 -> Cyclorotor Lookup Table/3
  Demux4/1 -> Mux/1
  Sum/1 -> Mux1/2
  Product/1 -> Sum/2
  Derivative/1 -> Product/1
  Constant1/1 -> Product/2

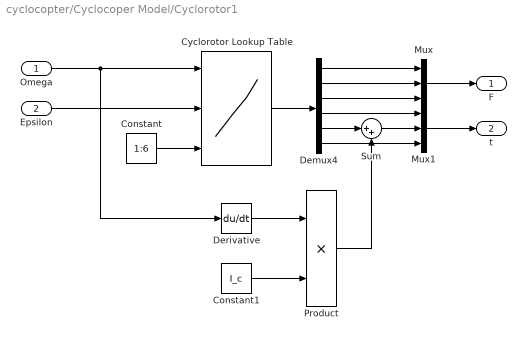
== system cyclocopter/Cyclocoper Model/Cyclorotor1 ==
  Omega : Inport
  Epsilon : Inport  Port=2
  Constant : Constant  Value=1:6
  Constant1 : Constant  Value=I_c
  Cyclorotor Lookup Table : Lookup_n-D  NumberOfTableDimensions=3  BreakpointsForDimension1=breakpoint_omega  BreakpointsForDimension2=breakpoint_epsilon  BreakpointsForDimension3=[1:6]  Table=cyclorotor_lookup  InternalRulePriority=Speed  OutDataTypeStr=double  RndMeth=Simplest  InputSameDT=on
  Demux4 : Demux  Outputs=6
  Derivative : Derivative
  Mux : Mux  Inputs=3
  Mux1 : Mux  Inputs=3
  Product : Product
  Sum : Sum  Inputs=|++
  F : Outport
  t : Outport  Port=2
  wires:
  Constant1/1 -> Product/2
  Derivative/1 -> Product/1
  Product/1 -> Sum/2
  Sum/1 -> Mux1/2
  Demux4/1 -> Mux/1
  Constant/1 -> Cyclorotor Lookup Table/3
  Demux4/2 -> Mux/2
  Demux4/3 -> Mux/3
  Demux4/6 -> Mux1/3
  Demux4/4 -> Mux1/1
  Demux4/5 -> Sum/1
  Mux1/1 -> t/1
  Omega/1 -> Cyclorotor Lookup Table/1, Derivative/1
  Epsilon/1 -> Cyclorotor Lookup Table/2
  Mux/1 -> F/1
  Cyclorotor Lookup Table/1 -> Demux4/1

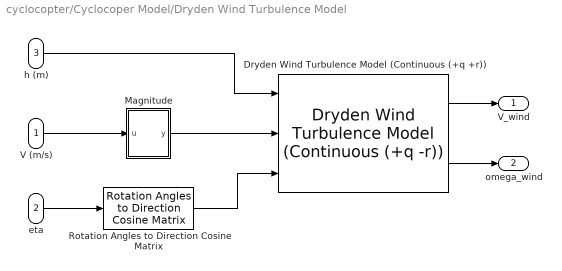
== system cyclocopter/Cyclocoper Model/Dryden Wind Turbulence Model ==
  V (m/s) : Inport
  eta : Inport  Port=2
  h (m) : Inport  Port=3
  Dryden Wind Turbulence Model (Continuous (+q +r)) : aerolibwind2/Dryden Wind Turbulence Model  (Continuous (+q -r))  units=Metric (MKS)  spec=MIL-F-8785C  model=Discrete Dryden (+q +r)  W20=ws  Wdeg=0  TurbProb=2x10^-1  L_high=533.4  Wingspan=0.5  ts=0.1  Seed=[23345 23346 23347 23348]  T_on=on
  Magnitude : MATLAB Function  TreatAsAtomicUnit=on
  Rotation Angles to Direction Cosine Matrix : aerolibtransform2/Rotation Angles to Direction Cosine Matrix  rotationOrder=XYZ
  V_wind : Outport
  omega_wind : Outport  Port=2
  wires:
  eta/1 -> Rotation Angles to Direction Cosine Matrix/1
  V (m/s)/1 -> Magnitude/1(u)
  Dryden Wind Turbulence Model (Continuous (+q +r))/2 -> omega_wind/1
  Dryden Wind Turbulence Model (Continuous (+q +r))/1 -> V_wind/1
  Rotation Angles to Direction Cosine Matrix/1 -> Dryden Wind Turbulence Model (Continuous (+q +r))/3
  Magnitude/1(y) -> Dryden Wind Turbulence Model (Continuous (+q +r))/2
  h (m)/1 -> Dryden Wind Turbulence Model (Continuous (+q +r))/1

== matlab function cyclocopter/Cyclocoper Model/MATLAB Function ==
  data: xi_dd output size=3; omega_d output size=3; eta_d output size=3; Fc1 input size=3; tc1 input size=3; Fc2 input size=3; tc2 input size=3; Fp input size=3; tp input size=3; oldStates input size=12
function [xi_dd, omega_d, eta_d] = fcn(Fc1, tc1, Fc2, tc2, Fp, tp,...
                                                   oldStates)

[xi_dd, omega_d, eta_d] = CyclocopterBody(Fc1, tc1, Fc2, tc2, Fp, tp,...
                                                   oldStates);

== matlab function cyclocopter/Cyclorotor Dual Limits ==
  data: val1 input; out1 output; val2 input; LL parameter; UL parameter; out2 output
function [out1, out2] = fcn(val1, val2, LL, UL)

dist = abs(val1 - val2); % calculate distance between values

% Setup outputs
out1 = val1;
out2 = val2;

% if strayed outside limits shift other value to compensate
if val1 > UL
    out2 = UL - dist;
elseif val1 < LL
    out2 = LL + dist;
elseif val2 > UL
    out1 = UL - dist;
elseif val2 < LL
    out1 = LL + dist;
end

% Cap outputs to upper and lower limits
if val1 > UL
    out1 = UL;
elseif val1 < LL
    out1 = LL;
end

if  val2 > UL
    out2 = UL;
elseif val2 < LL
    out2 = LL;
end

== matlab function cyclocopter/Servo Dual Limits ==
  data: val1 input; out1 output; val2 input; LL parameter; UL parameter; out2 output
function [out1, out2] = fcn(val1, val2, LL, UL)

dist = abs(val1 - val2); % calculate distance between values

% Setup outputs
out1 = val1;
out2 = val2;

% if strayed outside limits shift other value to compensate
if val1 > UL
    out2 = UL - dist;
elseif val1 < LL
    out2 = LL + dist;
elseif val2 > UL
    out1 = UL - dist;
elseif val2 < LL
    out1 = LL + dist;
end

% Cap outputs to upper and lower limits
if val1 > UL
    out1 = UL;
elseif val1 < LL
    out1 = LL;
end

if  val2 > UL
    out2 = UL;
elseif val2 < LL
    out2 = LL;
end

== matlab function cyclocopter/Cyclocoper Model/Dryden Wind Turbulence Model/Magnitude ==
  data: u input size=3; y output size=1
function y = fcn(u)
%#codegen

y = sqrt(u' * u);

== matlab function cyclocopter/Cyclocoper Model/Balancing Motor ==
  data: omega_p input; F_p output size=3; t_p output size=3; omega_p_d input; I_m parameter
% Balancing motor torque and force characteristics
function [F_p, t_p] = fcn(omega_p, omega_p_d, I_m)

t_p = [0; 0; 0];
F_p = [0; 0; 0];

if (omega_p > 0)

    w_p_RPM = omega_p * (60 / (2 * pi)); %          Convert from rad/s to RPM

    % From Motor_RPM_Characteristics curve fitting
    t = 1.176e-10 * w_p_RPM^2 -1.053e-07 * w_p_RPM + 0.003637;
    F = 4.773e-09 * w_p_RPM^2 -2.802e-06 * w_p_RPM - 0.002665;

    % Return vector
    F_p(3) = F;
    
    t_wp = omega_p_d * I_m;
    t_p(3) = -(t + t_wp);

    F_p = F_p * 10;
end
